simulink model "Codunction_180"  (R2021a)
settings: Solver=ode23s  StartTime=0.0  StopTime=.02*20  MaxStep=1e-6  RelTol=1e-3
libraries: spsIGBTDiodeLib x12, spsThreePhaseVIMeasurementLib x3, dsparch4 x2, spsDCVoltageSourceLib x2, spsRMSLib x2, simulink x2, spsSeriesRLCBranchLib x2, spsVoltageMeasurementLib x2, spsAsynchronousMachineSIUnitsLib x1, spsGroundLib x1, spsThreePhaseSeriesRLCBranchLib x1, spspowerguiLib x1
settings Model: Creator=20127  LastModifiedBy=Ahmed Mohamed
settings SolverCC: AlgebraicLoopSolver=TrustRegion
settings DataIOCC: ReturnWorkspaceOutputs=off
settings DebuggingCC: SFMachineParentedDataDiag=warning  ArithmeticOperatorsInVariantConditions=warning
settings SFSimCC: SimUseLocalCustomCode=off  CustomCodeUndefinedFunction=UseInterfaceOnly
settings RTWCC: RTWUseLocalCustomCode=off
settings CodeAppCC: StateflowObjectComments=on
settings SimscapeCC: SimscapeNormalizeSystem=off

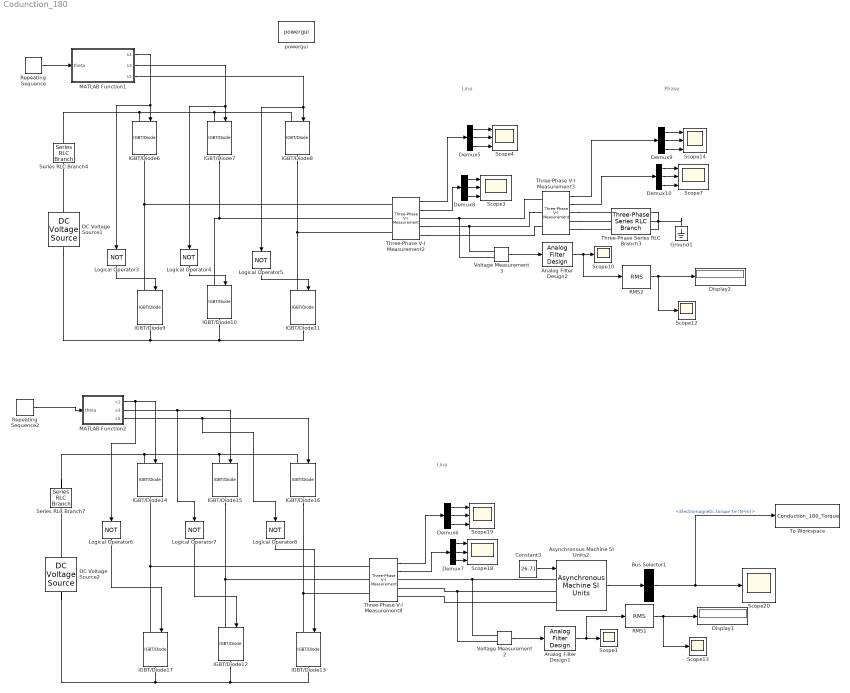
== system Codunction_180 ==
  note: Line
  note: Phase
  note: Line
  Analog Filter Design1 : dsparch4/Analog Filter Design  method=Butterworth  filttype=Lowpass  N=8  Wlo=2*pi*100  Whi=80  Rp=2  Rs=40
  Analog Filter Design2 : dsparch4/Analog Filter Design  method=Butterworth  filttype=Lowpass  N=3  Wlo=2*pi*100  Whi=80  Rp=2  Rs=40
  Asynchronous Machine SI Units2 : spsAsynchronousMachineSIUnitsLib/Asynchronous Machine SI Units  RotorType=Squirrel-cage  PresetModel="15:  5.4 HP (4KW)   400 V  50Hz 1430 RPM"  MechanicalLoad=Torque Tm  ShowDetailedParameters=on  ReferenceFrame=Rotor  Units=SI  MeasurementBus=off  NominalParameters=[4000 400 50]  VoltageRatio=1  Stator=[1.405 0.005839]  Rotor=[1.395 0.005839]  Cage1=[0.4155 0.002066]  Cage2=[0.4168 0.0003495]  Lm=0.1722  Mechanical=[0.0131 0.002985 2]  PolePairs=2  InitialConditions=[1 0 0 0 0 0 0 0]  SimulateSaturation=off  Saturation=[14.03593122, 27.81365428, 53.79336849, 72.68890987, 97.98006896, 148.6815601, 215.7428561, 302.9841135, 428.7778367 ; 230, 322, 414, 460, 506, 552, 598, 644, 690]  LoadFlowParameters=1492000  TsPowergui=0  TsBlock=-1  IterativeModel=Trapezoidal non iterative  IterativeDiscreteModel=Trapezoidal non iterative  Pmec=1.492e+006
  Bus Selector1 : BusSelector  OutputSignals=Mechanical.Electromagnetic torque Te (N*m)
  Constant3 : Constant  Value=26.71
  DC Voltage Source1 : spsDCVoltageSourceLib/DC Voltage Source  Amplitude=515  Measurements=None
  DC Voltage Source2 : spsDCVoltageSourceLib/DC Voltage Source  Amplitude=515  Measurements=None
  Demux{5..10} (6 alike) : Demux  Outputs=3
  Display1 : Display
  Display2 : Display
  Ground1 : spsGroundLib/Ground  LConnTagsString=a
  IGBT/Diode{6..17} (12 alike) : spsIGBTDiodeLib/IGBT//Diode  Ron=1e-3  Rs=1e5  Cs=inf  Measurements=off
  Logical Operator{3..8} (6 alike) : Logic  Operator=NOT  Inputs=1  AllPortsSameDT=off  OutDataTypeStr=boolean
  MATLAB Function1 : MATLAB Function  TreatAsAtomicUnit=on
  MATLAB Function2 : MATLAB Function  TreatAsAtomicUnit=on
  RMS1 : spsRMSLib/RMS  TrueRMS=off  Freq=50  RMSInit=0  Ts=0
  RMS2 : spsRMSLib/RMS  TrueRMS=off  Freq=50  RMSInit=0  Ts=0
  Repeating Sequence : simulink/Sources/Repeating Sequence  rep_seq_t=[0 0.02]  rep_seq_y=[0 2*pi]
  Repeating Sequence2 : simulink/Sources/Repeating Sequence  rep_seq_t=[0 0.02]  rep_seq_y=[0 2*pi]
  Scope{1,10,12..13,20} (5 alike) : Scope
  Scope{3..4,7,14,18..19} (6 alike) : Scope  NumInputPorts=3
  Series RLC Branch4 : spsSeriesRLCBranchLib/Series RLC Branch  LConnTagsString=__new0  RConnTagsString=__new0  BranchType=R  Resistance=0.1  Inductance=1e-3  SetiL0=off  InitialCurrent=0  Capacitance=1e-6  Setx0=off  InitialVoltage=0  Measurements=None
  Series RLC Branch7 : spsSeriesRLCBranchLib/Series RLC Branch  LConnTagsString=__new0  RConnTagsString=__new0  BranchType=R  Resistance=0.1  Inductance=1e-3  SetiL0=off  InitialCurrent=0  Capacitance=1e-6  Setx0=off  InitialVoltage=0  Measurements=None
  Three-Phase Series RLC Branch3 : spsThreePhaseSeriesRLCBranchLib/Three-Phase Series RLC Branch  LConnTagsString=A|B|C  RConnTagsString=A|B|C  BranchType=RL  Resistance=7.5*sqrt(2)  Inductance=7.5*sqrt(2)/314  Capacitance=1e-6  Measurements=None
  Three-Phase V-I Measurement2 : spsThreePhaseVIMeasurementLib/Three-Phase V-I Measurement  VoltageMeasurement=phase-to-phase  SetLabelV=off  LabelV=Vabc  Vpu=off  VpuLL=off  CurrentMeasurement=yes  SetLabelI=off  LabelI=Iabc  Ipu=off  Pbase=100e6  Vbase=500e3  OutputType=Complex  PhasorSimulation=off  PSBequivalent=0
  Three-Phase V-I Measurement3 : spsThreePhaseVIMeasurementLib/Three-Phase V-I Measurement  VoltageMeasurement=phase-to-ground  SetLabelV=off  LabelV=Vabc  Vpu=off  VpuLL=off  CurrentMeasurement=yes  SetLabelI=off  LabelI=Iabc  Ipu=off  Pbase=100e6  Vbase=500e3  OutputType=Complex  PhasorSimulation=off  PSBequivalent=0
  Three-Phase V-I Measurement8 : spsThreePhaseVIMeasurementLib/Three-Phase V-I Measurement  VoltageMeasurement=phase-to-phase  SetLabelV=off  LabelV=Vabc  Vpu=off  VpuLL=off  CurrentMeasurement=yes  SetLabelI=off  LabelI=Iabc  Ipu=off  Pbase=100e6  Vbase=500e3  OutputType=Complex  PhasorSimulation=off  PSBequivalent=0
  To Workspace : ToWorkspace  VariableName=Conduction_180_Torque  SampleTime=-1
      settings: Save2DSignal=2-D array (concatenate along first dimension)
  Voltage Measurement2 : spsVoltageMeasurementLib/Voltage Measurement  PhasorSimulation=off  OutputType=Complex  PSBequivalent=0
  Voltage Measurement3 : spsVoltageMeasurementLib/Voltage Measurement  PhasorSimulation=off  OutputType=Complex  PSBequivalent=0
  powergui : spspowerguiLib/powergui  Priority=1  SimulationMode=Continuous  SampleTime=50e-6  frequency=60  Iterations=50  frequencyindice=0  Pbase=100e6  ErrMax=1e-4  UnitsV=kV  UnitsW=MW  buscounter=0  FunctionMessages=off  echomessages=off  EnableUseOfTLC=off  CurrentSourceSwitches=off  DisableSnubberDevices=off  DisableRonSwitches=off  DisableVfSwitches=off  DisplayEquations=off  AutomaticDiscreteSolvers=off  SolverType=Tustin/Backward Euler (TBE)  Interpol=off  ExternalGateDelay=off  methode=off  Ts=10  x0status=blocks  SPID=off  SwTol=0  HookPort=off  NonlinearTolerance=1e-4  nMaxIteration=100  ContinueOnMaxIteration=off  RestoreLinks=warning  ResistiveCurrentMeasurement=off  Frange=[0:2:500]  Ylog=off  Xlog=on  ShowGrid=off  save=off  variable=ZData  structure=0  ZoomFFT=off  StartTime=0.0  cycles=1  DisplayStyle=1  fundamental=60  FreqAxis=off  MaxFrequency=1000  frequencyindicesteady=1  RmsSteady=1  display=off
  wires:
  Logical Operator3/1 -> IGBT/Diode9/1
  Logical Operator5/1 -> IGBT/Diode11/1
  Logical Operator4/1 -> IGBT/Diode10/1
  MATLAB Function1/3(s5) -> Logical Operator5/1, IGBT/Diode8/1
  MATLAB Function1/2(s3) -> Logical Operator4/1, IGBT/Diode7/1
  MATLAB Function1/1(s1) -> Logical Operator3/1, IGBT/Diode6/1
  Repeating Sequence/1 -> MATLAB Function1/1(theta)
  Repeating Sequence2/1 -> MATLAB Function2/1(theta)
  MATLAB Function2/1(s1) -> Logical Operator6/1, IGBT/Diode14/1
  MATLAB Function2/2(s3) -> Logical Operator7/1, IGBT/Diode15/1
  MATLAB Function2/3(s5) -> Logical Operator8/1, IGBT/Diode16/1
  Logical Operator7/1 -> IGBT/Diode12/1
  Logical Operator8/1 -> IGBT/Diode13/1
  Logical Operator6/1 -> IGBT/Diode17/1
  Three-Phase V-I Measurement3/1 -> Demux9/1
  Demux10/1 -> Scope7/1
  Voltage Measurement3/1 -> Analog Filter Design2/1
  Demux10/2 -> Scope7/2
  Three-Phase V-I Measurement2/1 -> Demux5/1
  Demux8/1 -> Scope3/1
  Three-Phase V-I Measurement3/2 -> Demux10/1
  Three-Phase V-I Measurement2/2 -> Demux8/1
  Demux5/2 -> Scope4/2
  Demux9/2 -> Scope14/2
  Demux8/2 -> Scope3/2
  Demux9/3 -> Scope14/3
  Demux9/1 -> Scope14/1
  Analog Filter Design2/1 -> Scope10/1, RMS2/1
  Demux8/3 -> Scope3/3
  Demux10/3 -> Scope7/3
  RMS2/1 -> Scope12/1, Display2/1
  Demux5/3 -> Scope4/3
  Demux5/1 -> Scope4/1
  Demux6/1 -> Scope19/1
  Analog Filter Design1/1 -> Scope1/1, RMS1/1
  Demux7/3 -> Scope18/3
  Demux6/2 -> Scope19/2
  Constant3/1 -> Asynchronous Machine SI Units2/1
  Voltage Measurement2/1 -> Analog Filter Design1/1
  Three-Phase V-I Measurement8/1 -> Demux6/1
  Three-Phase V-I Measurement8/2 -> Demux7/1
  Demux7/2 -> Scope18/2
  Demux7/1 -> Scope18/1
  RMS1/1 -> Scope13/1, Display1/1
  Demux6/3 -> Scope19/3
  Bus Selector1/1 -> To Workspace/1, Scope20/1  "<Electromagnetic torque Te (N*m)>"
  Asynchronous Machine SI Units2/1 -> Bus Selector1/1
  connections:
  Series RLC Branch4/LConn1 -- IGBT/Diode7/LConn1 -- IGBT/Diode8/LConn1 -- IGBT/Diode6/LConn1
  DC Voltage Source1/LConn1 -- IGBT/Diode10/RConn1 -- IGBT/Diode11/RConn1 -- IGBT/Diode9/RConn1
  IGBT/Diode9/LConn1 -- Three-Phase V-I Measurement2/LConn1 -- IGBT/Diode6/RConn1
  IGBT/Diode7/RConn1 -- IGBT/Diode10/LConn1 -- Three-Phase V-I Measurement2/LConn2
  IGBT/Diode8/RConn1 -- Three-Phase V-I Measurement2/LConn3 -- IGBT/Diode11/LConn1
  DC Voltage Source1/RConn1 -- Series RLC Branch4/RConn1
  IGBT/Diode15/LConn1 -- IGBT/Diode16/LConn1 -- Series RLC Branch7/LConn1 -- IGBT/Diode14/LConn1
  IGBT/Diode12/RConn1 -- DC Voltage Source2/LConn1 -- IGBT/Diode17/RConn1 -- IGBT/Diode13/RConn1
  IGBT/Diode15/RConn1 -- Three-Phase V-I Measurement8/LConn2 -- IGBT/Diode12/LConn1
  IGBT/Diode16/RConn1 -- Three-Phase V-I Measurement8/LConn3 -- IGBT/Diode13/LConn1
  DC Voltage Source2/RConn1 -- Series RLC Branch7/RConn1
  IGBT/Diode17/LConn1 -- Three-Phase V-I Measurement8/LConn1 -- IGBT/Diode14/RConn1
  Ground1/LConn1 -- Three-Phase Series RLC Branch3/RConn2 -- Three-Phase Series RLC Branch3/RConn3 -- Three-Phase Series RLC Branch3/RConn1
  Three-Phase V-I Measurement3/LConn2 -- Three-Phase V-I Measurement2/RConn2 -- Voltage Measurement3/LConn1
  Three-Phase V-I Measurement2/RConn1 -- Three-Phase V-I Measurement3/LConn1 -- Voltage Measurement3/LConn2
  Three-Phase V-I Measurement3/RConn2 -- Three-Phase Series RLC Branch3/LConn2
  Three-Phase V-I Measurement3/RConn1 -- Three-Phase Series RLC Branch3/LConn1
  Three-Phase V-I Measurement3/RConn3 -- Three-Phase Series RLC Branch3/LConn3
  Three-Phase V-I Measurement2/RConn3 -- Three-Phase V-I Measurement3/LConn3
  Three-Phase V-I Measurement8/RConn2 -- Asynchronous Machine SI Units2/LConn2 -- Voltage Measurement2/LConn2
  Three-Phase V-I Measurement8/RConn1 -- Asynchronous Machine SI Units2/LConn1 -- Voltage Measurement2/LConn1
  Asynchronous Machine SI Units2/LConn3 -- Three-Phase V-I Measurement8/RConn3

== matlab function Codunction_180/MATLAB Function2 ==
  data: theta input; s1 output; s3 output; s5 output
function [s1 , s3 , s5 ] = fcn(theta)
if (theta >= 0) && (theta < pi/3 ) 
    s1 = 1 ;
    s3 = 0 ;
    s5 = 1 ;
elseif (theta >= pi/3 ) && (theta < 2*pi/3 ) 
    s1 = 1 ;
    s3 = 0 ;
    s5 = 0 ;
elseif (theta >= 2*pi/3 ) && (theta < pi ) 
    s1 = 1 ;
    s3 = 1 ;
    s5 = 0 ;
elseif (theta >= pi ) && (theta < 4*pi/3 ) 
    s1 = 0 ;
    s3 = 1 ;
    s5 = 0 ;
elseif (theta >= 4*pi/3 ) && (theta < 5*pi/3 ) 
    s1 = 0 ;
    s3 = 1 ;
    s5 = 1 ;
elseif (theta >= 5*pi/3 ) && (theta <= 2*pi ) 
    s1 = 0 ;
    s3 = 0 ;
    s5 = 1 ;
else 
s1 = 0 ;
s3 = 0 ;
s5 = 0 ;
end

== matlab function Codunction_180/MATLAB Function1 ==
  data: theta input; s1 output; s3 output; s5 output
function [s1 , s3 , s5 ] = fire_switches(theta)
if (theta >= 0) && (theta < pi/3 ) 
    s1 = 1 ;
    s3 = 0 ;
    s5 = 1 ;
elseif (theta >= pi/3 ) && (theta < 2*pi/3 ) 
    s1 = 1 ;
    s3 = 0 ;
    s5 = 0 ;
elseif (theta >= 2*pi/3 ) && (theta < pi ) 
    s1 = 1 ;
    s3 = 1 ;
    s5 = 0 ;
elseif (theta >= pi ) && (theta < 4*pi/3 ) 
    s1 = 0 ;
    s3 = 1 ;
    s5 = 0 ;
elseif (theta >= 4*pi/3 ) && (theta < 5*pi/3 ) 
    s1 = 0 ;
    s3 = 1 ;
    s5 = 1 ;
elseif (theta >= 5*pi/3 ) && (theta <= 2*pi ) 
    s1 = 0 ;
    s3 = 0 ;
    s5 = 1 ;
else 
s1 = 0 ;
s3 = 0 ;
s5 = 0 ;
end
